simulink model "IV_HeatConductionThroughIronRodLumped"  (R2024b)
settings: Solver=VariableStepAuto  StartTime=0.0  StopTime=2500  MaxStep=100  RelTol=1e-3  AbsTol=1e-3  EnableMultiTasking=on
PreLoadFcn:
  | if ~exist('D', 'var')         D= 0.025;       end % [m]
  | if ~exist('L', 'var')         L= 0.2;         end % [m]
  | if ~exist('A', 'var')         A= pi*D^2/4;    end % [m^2]
  | if ~exist('A_cyl', 'var')     A_cyl= pi*D*L;  end % [m^2]
  | if ~exist('k', 'var')         k= 80.2;        end % [W/(K*m)]
  | if ~exist('h', 'var')         h= 32.1;        end % [W/(K*m)]
  | if ~exist('m', 'var')         m= 7800*A*L;    end % [kg]
  | if ~exist('c', 'var')         c= 447;         end % [J/kg/K]
  | if ~exist('T_air', 'var')     T_air= 20;      end % [degC]
  | if ~exist('T_base', 'var')    T_base= 100;    end % [degC]
  | if ~exist('T_init', 'var')    T_init= 20;     end % [degC]
undefined symbols (not defined in the file): L, T_init
libraries: fl_lib x9, nesl_utility x3
Description:
  | Heat Conduction Through Iron Rod Using Lumped Mass
settings Model: Creator=The MathWorks, Inc.  LastModifiedBy=mvahab
settings SolverCC: AutoScaleAbsTol=off  AlgebraicLoopSolver=TrustRegion
settings DataIOCC: LimitDataPoints=on  SaveFormat=Array  ReturnWorkspaceOutputs=off  TimeSaveName=tout_lumped_mass_model  OutputSaveName=yout_lumped_mass_model
settings OptimizationCC: LifeSpan=inf
settings DebuggingCC: SolverPrmCheckMsg=warning  UnconnectedInputMsg=warning  UnconnectedOutputMsg=warning  UnconnectedLineMsg=warning  AllowSymbolicDim=off  PregeneratedLibrarySubsystemCodeDiagnostic=none  SFUnexpectedBacktrackingDiag=warning  SFNoUnconditionalDefaultTransitionDiag=warning  SFExecutionAtInitializationDiag=none  ArithmeticOperatorsInVariantConditions=warning
settings HardwareCC: ProdBitPerPointer=32  ProdBitPerSizeT=32  ProdBitPerPtrDiffT=32  ProdLargestAtomicFloat=None  ProdIntDivRoundTo=Undefined  ProdEndianess=Unspecified  ProdWordSize=32  ProdHWDeviceType=32-bit Generic
settings ModelReferenceCC: EnableRefExpFcnMdlSchedulingChecks=on  PropagateSignalLabelsOutOfModel=off
settings SFSimCC: SimUseLocalCustomCode=off  CustomCodeUndefinedFunction=UseInterfaceOnly
settings RTWCC: RTWUseLocalCustomCode=off  GPUComputeCapability=3.5  DLArmComputeVersion=19.05
settings CodeAppCC: StateflowObjectComments=on
settings GRTTargetCC: TargetLangStandard=C89/C90 (ANSI)
settings ConfigComp: CovMetricSettings=dw  CovSaveCumulativeToWorkspaceVar=on  CovSaveSingleToWorkspaceVar=on  CovExternalEMLEnable=off  CovSFcnEnable=off
settings SimscapeCC: SimscapeLogType=all  SimscapeLogSimulationStatistics=on  SimscapeLogName=simlog_HeatConductionThroughIronRodLumped  SimscapeLogDataHistory=10000

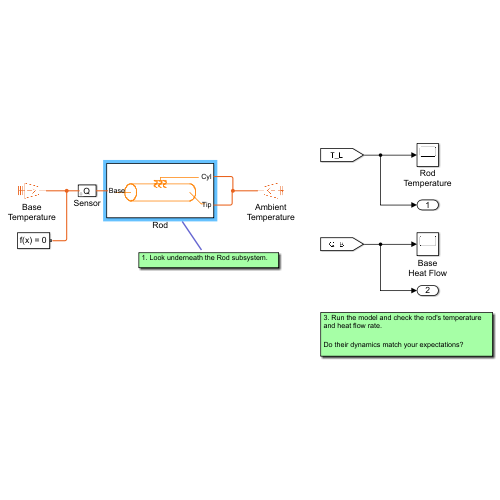
[thumbnail: Simulink's stored preview of the top-level diagram]
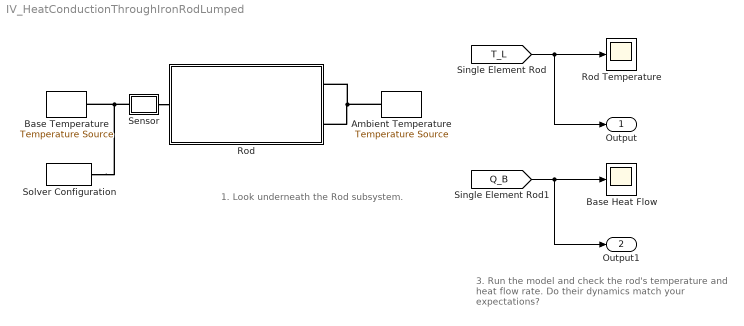
== system IV_HeatConductionThroughIronRodLumped ==
  note: 1. Look underneath the Rod subsystem.
  note: 3. Run the model and check the rod's temperature and heat flow rate.
      |
      | Do their dynamics match your expectations?
  Ambient Temperature : fl_lib/Thermal/Thermal Sources/Temperature Source  temperature=T_air degC
  Base Heat Flow : Scope
  Base Temperature : fl_lib/Thermal/Thermal Sources/Temperature Source  temperature=T_base degC
  Rod : Subsystem
      mask Display:
      | color('orange');
      | 
      | % Plot cylinder
      | plot([1,3],[1,1])
      | plot([1,3],[2,2])
      | plot(0.2*cos(0:2*pi/500:2*pi)+1,0.5*sin(0:2*pi/500:2*pi)+1.5)
      | plot(0.2*cos(-pi/2:2*pi/500:pi/2)+3,0.5*sin(-pi/2:2*pi/500:pi/2)+1.5)
      | 
      | % Heat Port
      | plot([1.8 2.2],[2.2 2.2])
      | plot([0.1*cos(-pi/2:0.1:pi/2)+1.8],[0.1*sin(-pi/2:0.1:pi/2)+2.1])
      | plot([0.1*cos(pi/2:0.1:3*pi/2)+1.9],[0.1*sin(pi/2:0.1:3*pi/2)+1.9])
      | plot([0.1*cos(-pi/2:0.1:pi/2)+1.95],[0.1*sin(-pi/2:0.1:pi/2)+2.1])
      | plot([0.1*cos(pi/2:0.1:3*pi/2)+2.05],[0.1*sin(pi/2:0.1:3*pi/2)+1.9])
      | plot([0.1*cos(-pi/2:0.1:pi/2)+2.1],[0.1*sin(-pi/2:0.1:pi/2)+2.1])
      | plot([0.1*cos(pi/2:0.1:3*pi/2)+2.2],[0.1*sin(pi/2:0.1:3*pi/2)+1.9])
      | 
      | % Connecting lines
      | plot([2 3.3],[2.4,2.4])
      | plot([2 2],[2.2 2.4])
      | plot([0.5 1],[1.5 1.5])
      | plot([3.4 3.5],[0.8 0.8])
      | plot([3,3.4],[1.5 0.8])
      | % Scaling
      | color('white')
      | plot(0.2,0)
      | plot(3.8,3.2)
  Rod Temperature : Scope
  Sensor : Subsystem
      mask Display: fprintf('Q')
  Solver Configuration : nesl_utility/Solver Configuration  PhysicalDomain=network_engine_domain  SubClassName=solver  LeftPortType=input  RightPortType=generic  Tones=[]  Harmonics=[]  SimulateNoise=off  Profile=off  UseLocalSampling=off  EnableSwitchedLinearOptims=on  FrequencyDomain=off  UseCCode=off  RelTol=0.001  AbsTol=1e-06  MinStep=1e-09  ToWorkspace=off  RevertToSquareIcSolve=off  NumHomotopyIterations=100  PhasorMode=off  PhasorModeNumHarmonics=1  ConsistencySolver=NEWTON_XTOL_AFTER_FTOL  IndexReductionMethod=DerivativeReplacement  DoDC=off  ResidualTolerance=1e-9  ConsistencyTolSource=GLOBAL  ConsistencyAbsTol=0.001  ConsistencyRelTol=0.001  ConsistencyTolFactor=0.001  UseLocalSolver=off  LocalSolverChoice=NE_BACKWARD_EULER_ADVANCER  ResolveIndetEquations=on  FunctionEvalNumThread=1  LocalSolverSampleTime=.001  DoFixedCost=off  MaxNonlinIter=3  MaxModeIter=2  ComputeImpulses=off  ImpulseIterations=2  LinearAlgebra=auto  LinearAlgebraNumThread=0  EquationFormulation=NE_TIME_EF  DelaysMemoryBudget=1024  AutomaticFiltering=on  FilteringTimeConstant=0.001  PartitionStorageMethod=AS_NEEDED  PartitionMemoryBudget=1024  PartitionMethod=FAST  MultibodyUseLocalSolver=off  MultibodyLocalSolverChoice=ODE1  MultibodyLocalSolverSampleTime=0.001
  Output : Outport
  Output1 : Outport  Port=2
  wires:
  [T_L] -> Output/1, Rod Temperature/1
  [Q_B] -> Output1/1, Base Heat Flow/1
  connections:
  Ambient Temperature/LConn1 -- Rod/RConn1 -- Rod/RConn2
  Sensor/RConn1 -- Rod/LConn1
  Sensor/LConn1 -- Solver Configuration/RConn1 -- Base Temperature/LConn1

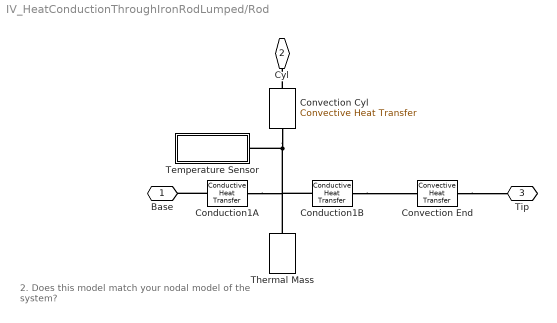
== system IV_HeatConductionThroughIronRodLumped/Rod ==
  note: 2. Does this model match your nodal model of the system?
  Conduction1A : fl_lib/Thermal/Thermal Elements/Conductive Heat Transfer  thermal_type=foundation.enum.ConstantVariableTabulated.Constant  wall_geometry=foundation.enum.ConductionWallGeometry.Planar  area=A m^2  thickness=L/2 m  d_in=0.05 m  d_out=0.1 m  L=1 m  th_cond_min=10 W/(K*m)  th_cond=k W/(m*K)  th_cond_TLU=[413, 401, 392, 383, 371, 357, 342] W/(K*m)  temp_TLU=[200, 273, 400, 600, 800, 1000, 1200] K  T_specify=off  T_priority=None  T=0 K  T_nominal_specify=off  T_nominal_value=1  T_nominal_unit=K  Q_specify=off  Q_priority=None  Q=0 W  Q_nominal_specify=off  Q_nominal_value=1  Q_nominal_unit=W
  Conduction1B : fl_lib/Thermal/Thermal Elements/Conductive Heat Transfer  thermal_type=foundation.enum.ConstantVariableTabulated.Constant  wall_geometry=foundation.enum.ConductionWallGeometry.Planar  area=A m^2  thickness=L/2 m  d_in=0.05 m  d_out=0.1 m  L=1 m  th_cond_min=10 W/(K*m)  th_cond=k W/(m*K)  th_cond_TLU=[413, 401, 392, 383, 371, 357, 342] W/(K*m)  temp_TLU=[200, 273, 400, 600, 800, 1000, 1200] K  T_specify=off  T_priority=None  T=0 K  T_nominal_specify=off  T_nominal_value=1  T_nominal_unit=K  Q_specify=off  Q_priority=None  Q=0 W  Q_nominal_specify=off  Q_nominal_value=1  Q_nominal_unit=W
  Convection Cyl : fl_lib/Thermal/Thermal Elements/Convective Heat Transfer  thermal_type=foundation.enum.constant_variable.constant  area=A_cyl m^2  heat_tr_coeff=h W/(m^2 * K)  min_heat_tr_coeff=1e-3 W/(K*m^2)  T_specify=off  T_priority=None  T=0 K  T_nominal_specify=off  T_nominal_value=1  T_nominal_unit=K  Q_specify=off  Q_priority=None  Q=0 W  Q_nominal_specify=off  Q_nominal_value=1  Q_nominal_unit=W
  Convection End : fl_lib/Thermal/Thermal Elements/Convective Heat Transfer  thermal_type=foundation.enum.constant_variable.constant  area=A m^2  heat_tr_coeff=h W/(m^2 * K)  min_heat_tr_coeff=1e-3 W/(K*m^2)  T_specify=off  T_priority=None  T=0 K  T_nominal_specify=off  T_nominal_value=1  T_nominal_unit=K  Q_specify=off  Q_priority=None  Q=0 W  Q_nominal_specify=off  Q_nominal_value=1  Q_nominal_unit=W
  Temperature Sensor : Subsystem
  Thermal Mass : fl_lib/Thermal/Thermal Elements/Thermal Mass  mass_type=foundation.enum.constant_variable.constant  mass=m kg  sp_heat=c J/kg/K  mass_min=1e-6 kg  num_ports=foundation.enum.numPorts2.one  m_specify=off  m_priority=High  m=1 kg  m_nominal_specify=off  m_nominal_value=1  m_nominal_unit=kg  T_specify=on  T_priority=High  T=T_init degC  T_nominal_specify=off  T_nominal_value=1  T_nominal_unit=K  Q_specify=off  Q_priority=None  Q=0 W  Q_nominal_specify=off  Q_nominal_value=1  Q_nominal_unit=W
  Base : PMIOPort  Side=Left
  Cyl : PMIOPort  Port=2  Side=Right
  Tip : PMIOPort  Port=3  Side=Right
  connections:
  Conduction1A/LConn1 -- Base/RConn1
  Convection Cyl/RConn1 -- Cyl/RConn1
  Conduction1B/RConn1 -- Convection End/LConn1
  Conduction1A/RConn1 -- Conduction1B/LConn1 -- Thermal Mass/LConn1 -- Convection Cyl/LConn1 -- Temperature Sensor/LConn1
  Convection End/RConn1 -- Tip/RConn1

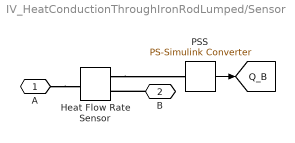
== system IV_HeatConductionThroughIronRodLumped/Sensor ==
  Heat Flow Rate Sensor : fl_lib/Thermal/Thermal Sensors/Heat Flow Rate Sensor
  PSS : nesl_utility/PS-Simulink Converter  PhysicalDomain=network_engine_domain  SubClassName=ps_output  LeftPortType=input  RightPortType=output  PseudoPeriodic=off  Frequencies=[]  VectorFormat=1-D array  Unit=W  AffineConversion=off
  A : PMIOPort  Side=Left
  B : PMIOPort  Port=2  Side=Right
  tag scope: Q_B=global
  wires:
  PSS/1 -> [Q_B]
  connections:
  A/RConn1 -- Heat Flow Rate Sensor/LConn1
  B/RConn1 -- Heat Flow Rate Sensor/RConn2
  Heat Flow Rate Sensor/RConn1 -- PSS/LConn1

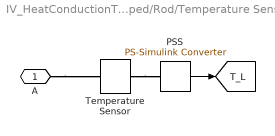
== system IV_HeatConductionThroughIronRodLumped/Rod/Temperature Sensor ==
  PSS : nesl_utility/PS-Simulink Converter  PhysicalDomain=network_engine_domain  SubClassName=ps_output  LeftPortType=input  RightPortType=output  PseudoPeriodic=off  Frequencies=[]  VectorFormat=1-D array  Unit=degC  AffineConversion=on
  Temperature Sensor : fl_lib/Thermal/Thermal Sensors/Temperature Sensor  temperature_measure=foundation.enum.MeasurementReference.absolute
      settings: InternalSimscapePortConfiguration="{\"Bottom\":[],\"Left\":[{\"id\":\"A\",\"label\":\"A\",\"type\":\"foundation.thermal.thermal\"}],\"Right\":[{\"id\":\"T\",\"label\":\"T\",\"type\":\"output\"}],\"Top\":[]}"
  A : PMIOPort  Side=Left
  tag scope: T_L=global
  wires:
  PSS/1 -> [T_L]
  connections:
  A/RConn1 -- Temperature Sensor/LConn1
  Temperature Sensor/RConn1 -- PSS/LConn1
